simulink model "ChildsPhone"  (R2023a)
settings: Solver=FixedStepAuto  StartTime=0.0  StopTime=inf  RelTol=1e-3
undefined symbols (not defined in the file): DiscIntNeverNeededParam
libraries: androidaudiovideolib x4, androidcommunicationlib x4, androidsensorlib x3, androiduilib x2
settings Model: Creator=ketha  LastModifiedBy=ketha
settings OptimizationCC: EnhancedBackFolding=on  PassReuseOutputArgsAs=Individual arguments  ZeroExternalMemoryAtStartup=off  ZeroInternalMemoryAtStartup=off  MaxStackSize=64  OptimizeBlockOrder=speed  DifferentSizesBufferReuse=on  OptimizationCustomize=off  EfficientTunableParamExpr=on
settings DebuggingCC: ParameterTunabilityLossMsg=error  UnderSpecifiedDimensionMsg=warning
settings HardwareCC: ProdBitPerPointer=32  ProdBitPerSizeT=32  ProdBitPerPtrDiffT=32  ProdLargestAtomicInteger=Long  ProdLargestAtomicFloat=Double  ProdWordSize=32  ProdHWDeviceType=ARM Compatible->ARM Cortex
settings SFSimCC: MATLABDynamicMemAlloc=off
settings RTWCC: Description=Embedded Coder  SystemTargetFile=ert.tlc  HardwareBoard=Android Device  TLCOptions="-aInlineSetEventsForThisBaseRateFcn=TLC_FALSE -aSuppressMultiTaskScheduler=TLC_FALSE  -aRateBasedStepFcn=0"  TemplateMakefile=ert_default_tmf  RTWVerbose=off  Toolchain=Android SDK/NDK Tools  BuildConfiguration=Faster Runs
settings CodeAppCC: ForceParamTrailComments=on  IgnoreCustomStorageClasses=off  OperatorAnnotations=on  SimulinkDataObjDesc=on  SFDataObjDesc=on  InsertBlockDesc=on
settings ERTTargetCC: SupportContinuousTime=on

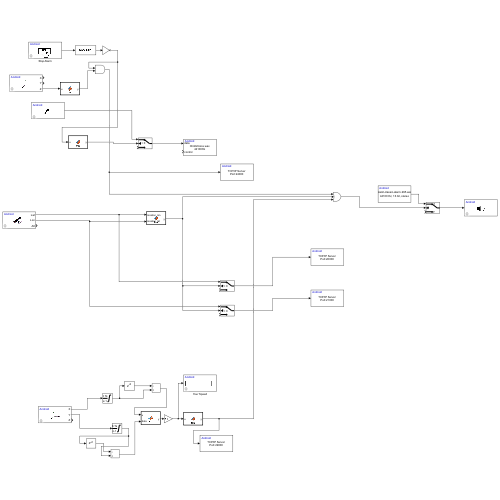
[thumbnail: Simulink's stored preview of the top-level diagram]
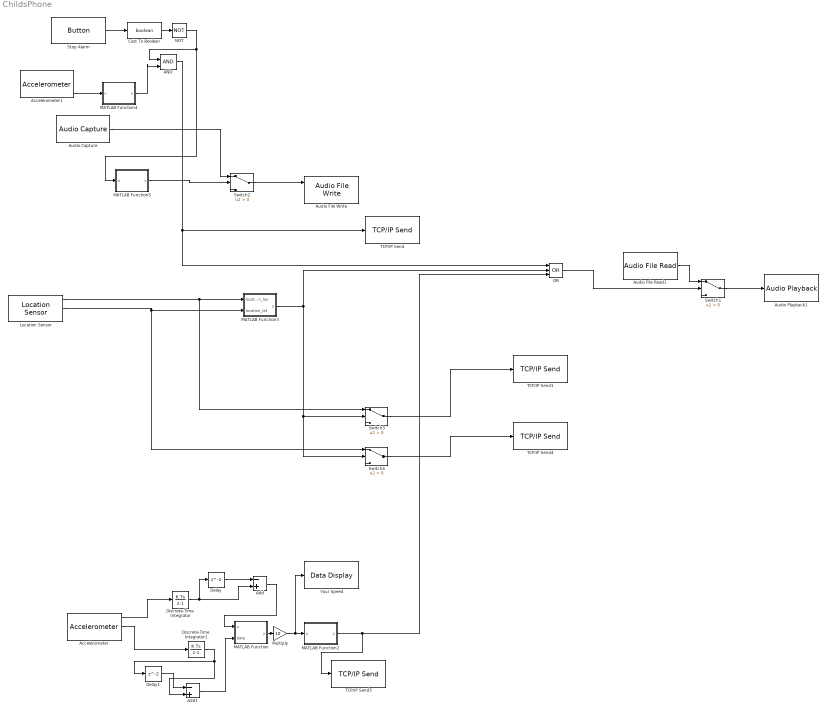
== system ChildsPhone ==
  AND : Logic  IconShape=distinctive  AllPortsSameDT=off  OutDataTypeStr=boolean
  Accelerometer : androidsensorlib/Accelerometer  OutputVector=off  SampleTime=0.1  BlockPlatform=Android
  Accelerometer1 : androidsensorlib/Accelerometer  OutputVector=off  SampleTime=0.1  BlockPlatform=Android
  Add : Sum  Inputs=-+
  Add1 : Sum  Inputs=-+
  Audio Capture : androidaudiovideolib/Audio Capture  SampleFreq=44100  FrameSize=4410  SampleTime=0.1  SimulateUsing=Code generation  DeviceStr=0  QueueDuration=0  BlockPlatform=Android  AudioSamplingFreq=44100
  Audio File Read1 : androidaudiovideolib/Audio File Read  FileName=C:\Users\ketha\OneDrive\Desktop\Darshan_c\Darshan_SSRP\mixkit-classic-alarm-995.wav  FrameSize=4410
  Audio File Write : androidaudiovideolib/Audio File Write  FileName=ChildsVoice  FileType=wav  AudioSamplingFreq=44100  RecordTimeControl=Input port  MaxRecordTime=60  BitRate=128  AudioFileWriteId=ChildsPhone/Audio_File_Write
  Audio Playback1 : androidaudiovideolib/Audio Playback  SampleFreq=44100  AudioSamplingFreq=44100  SampleTime=0.1  DeviceStr=0  QueueDuration=0  BlockPlatform=Android
  Cast To Boolean : DataTypeConversion  OutDataTypeStr=boolean  SaturateOnIntegerOverflow=off  RndMeth=Floor
  Delay : Delay
  Delay1 : Delay
  Discrete-Time Integrator : DiscreteIntegrator  SampleTime=0.1  LimitOutput=on  UpperSaturationLimit=100  LowerSaturationLimit=0  ICPrevOutput=DiscIntNeverNeededParam  ICPrevScaledInput=DiscIntNeverNeededParam
  Discrete-Time Integrator1 : DiscreteIntegrator  SampleTime=0.1  LimitOutput=on  UpperSaturationLimit=100  LowerSaturationLimit=0  ICPrevOutput=DiscIntNeverNeededParam  ICPrevScaledInput=DiscIntNeverNeededParam
  Location Sensor : androidsensorlib/Location Sensor  OutputVector=off  SampleTime=0.1  BlockPlatform=Android
  MATLAB Function : MATLAB Function  TreatAsAtomicUnit=on
  MATLAB Function2 : MATLAB Function  TreatAsAtomicUnit=on
  MATLAB Function3 : MATLAB Function  TreatAsAtomicUnit=on
  MATLAB Function4 : MATLAB Function  TreatAsAtomicUnit=on
  MATLAB Function5 : MATLAB Function  TreatAsAtomicUnit=on
  Multiply : Gain  Gain=10
  NOT : Logic  Operator=NOT  IconShape=distinctive  AllPortsSameDT=off  OutDataTypeStr=boolean
  OR : Logic  Operator=OR  Inputs=3  IconShape=distinctive  AllPortsSameDT=off  OutDataTypeStr=boolean
  Stop Alarm : androiduilib/Button  ButtonState=Not pressed  ButtonId=ChildsPhone/Stop_Alarm  State=off  SampleTime=0.1  BlockPlatform=Android
  Switch{1..4} (4 alike) : Switch  Criteria=u2 > Threshold  SaturateOnIntegerOverflow=off  InputSameDT=off
  TCP/IP Send : androidcommunicationlib/TCP//IP Send  TCPSendId=ChildsPhone/TCP//IP_Send  Mode_=Server  LocalServerPort_=24000  RemoteAddr_=127.0.0.1  RemoteServerPort_=25000  ClientPortBindingSelection_=off  ClientPortToBind_=35000  BlockingMode_=off  BlockTimeout_=0.1
  TCP/IP Send1 : androidcommunicationlib/TCP//IP Send  TCPSendId=ChildsPhone/TCP//IP_Send1  Mode_=Server  LocalServerPort_=26000  RemoteAddr_=127.0.0.1  RemoteServerPort_=25000  ClientPortBindingSelection_=off  ClientPortToBind_=35000  BlockingMode_=off  BlockTimeout_=0.1
  TCP/IP Send4 : androidcommunicationlib/TCP//IP Send  TCPSendId=ChildsPhone/TCP//IP_Send4  Mode_=Server  LocalServerPort_=21000  RemoteAddr_=127.0.0.1  RemoteServerPort_=25000  ClientPortBindingSelection_=off  ClientPortToBind_=35000  BlockingMode_=off  BlockTimeout_=0.1
  TCP/IP Send5 : androidcommunicationlib/TCP//IP Send  TCPSendId=ChildsPhone/TCP//IP_Send5  Mode_=Server  LocalServerPort_=29000  RemoteAddr_=127.0.0.1  RemoteServerPort_=25000  ClientPortBindingSelection_=off  ClientPortToBind_=35000  BlockingMode_=off  BlockTimeout_=0.1
  Your Speed : androiduilib/Data Display  DataDisplayId=ChildsPhone/Your_Speed  Format=Float  Precision=6  SimulateUsing=Code generation  blockPlatform=Android
  wires:
  Location Sensor/1 -> Switch3/1, MATLAB Function3/1(location_lon)
  NOT/1 -> MATLAB Function5/1(u), AND/1
  Accelerometer1/3 -> MATLAB Function4/1(u)
  MATLAB Function5/1(y) -> Switch2/2
  Stop Alarm/1 -> Cast To Boolean/1
  MATLAB Function4/1(y) -> AND/2
  Cast To Boolean/1 -> NOT/1
  Audio File Read1/1 -> Switch1/1
  Switch1/1 -> Audio Playback1/1
  AND/1 -> TCP/IP Send/1, OR/1
  OR/1 -> Switch1/2
  Location Sensor/2 -> Switch4/1, MATLAB Function3/2(location_lat)
  MATLAB Function3/1(y) -> Switch4/2, Switch3/2, OR/2
  Switch3/1 -> TCP/IP Send1/1
  Switch4/1 -> TCP/IP Send4/1
  Delay1/1 -> Add1/1
  Multiply/1 -> MATLAB Function2/1(u), Your Speed/1
  MATLAB Function/1(y) -> Multiply/1
  Accelerometer/1 -> Discrete-Time Integrator/1
  Discrete-Time Integrator/1 -> Delay/1, Add/2
  Add/1 -> MATLAB Function/1(u)
  Add1/1 -> MATLAB Function/2(data)
  Discrete-Time Integrator1/1 -> Add1/2, Delay1/1
  Accelerometer/2 -> Discrete-Time Integrator1/1
  Delay/1 -> Add/1
  MATLAB Function2/1(y) -> TCP/IP Send5/1, OR/3
  Audio Capture/1 -> Switch2/1
  Switch2/1 -> Audio File Write/1

== matlab function ChildsPhone/MATLAB Function2 ==
  data: u input; y output
function y = fcn(u)

% Specify y as single data type
y = single(u);

if u > 10
    y = single(1); % Use single() to specify the data type
else
    y = single(0); % Use single() to specify the data type
end

== matlab function ChildsPhone/MATLAB Function3 ==
  data: location_lon input; y output; location_lat input
function y = fcn(location_lon, location_lat)
    % Convert latitude and longitude from degrees to radians
    location_lat = deg2rad(location_lat);
    location_lon = deg2rad(location_lon);
    center_lat = deg2rad(23.209632);
    center_lon = deg2rad(72.683626);

    % Earth radius in meters
    earth_radius = 6371000; % Approximate value for the Earth's radius

    % Calculate the distance between the two points using Haversine formula
    dlat = location_lat - center_lat;
    dlon = location_lon - center_lon;
    a = sin(dlat/2)^2 + cos(center_lat) * cos(location_lat) * sin(dlon/2)^2;
    c = 2 * asin(min(1, sqrt(a)));

    distance =50*c;

    % Check if the distance is within the radius
    if distance <=   49.182300% radius in meters
        y = single(0); % Location is inside the boundary
    else
        y = single(1); % Location is outside the boundary
    end
end

== matlab function ChildsPhone/MATLAB Function4 ==
  data: u input; y output
function y = fcn(u)

% Specify y as single data type
y = single(u);

if u < 4
    y = single(1); % Use single() to specify the data type
else
    y = single(0); % Use single() to specify the data type
end

== matlab function ChildsPhone/MATLAB Function5 ==
  data: u input; y output
function y = fcn(u)

if u == 0
    y = 1;
else
    y = 0;
end

== matlab function ChildsPhone/MATLAB Function ==
  data: u input; y output; data input
function y = fcn(u, data)

y = (u^2+data^2)^1/2;
